simulink model "imu"  (R2013b)
settings: Solver=ode3  StartTime=0.0  StopTime=20  FixedStep=0.001  RelTol=1e-3
undefined symbols (not defined in the file or in its folder): DiscIntNeverNeededParam
libraries: simulink x1
settings Model: Creator=Ugo Pattacini  LastModifiedBy=Ugo Pattacini

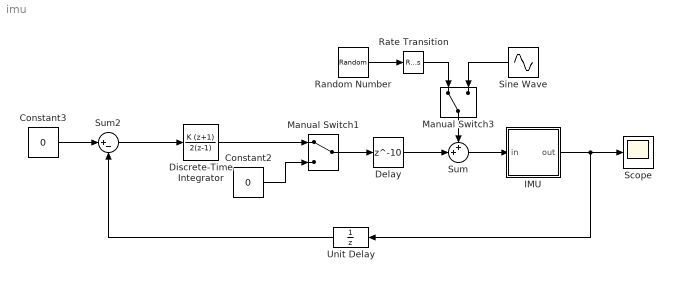
== system imu ==
  Constant2 : Constant  Value=0
  Constant3 : Constant  Value=0
  Delay : Delay  DelayLength=10  SampleTime=0.01
  Discrete-Time Integrator : DiscreteIntegrator  IntegratorMethod=Accumulation: Trapezoidal  gainval=0.05  SampleTime=0.01  ICPrevOutput=DiscIntNeverNeededParam  ICPrevScaledInput=DiscIntNeverNeededParam
  IMU : Subsystem
      mask Display: disp('IMU');
  Manual Switch1 : ManualSwitch
  Manual Switch3 : ManualSwitch
  Random Number : RandomNumber  Variance=20  SampleTime=2
  Rate Transition : RateTransition
  Scope : Scope
      settings: YMin=-20  YMax=20
  Sine Wave : Sin  Amplitude=20  Frequency=2*pi  SampleTime=0.01
  Sum : Sum  Inputs=++|  SampleTime=0.01
  Sum2 : Sum  Inputs=|+-
  Unit Delay : UnitDelay  SampleTime=-1
  wires:
  Constant2/1 -> Manual Switch1/2
  Sum2/1 -> Discrete-Time Integrator/1
  Constant3/1 -> Sum2/1
  Discrete-Time Integrator/1 -> Manual Switch1/1
  Unit Delay/1 -> Sum2/2
  Manual Switch3/1 -> Sum/1
  Random Number/1 -> Rate Transition/1
  Sine Wave/1 -> Manual Switch3/2
  Manual Switch1/1 -> Delay/1
  Delay/1 -> Sum/2
  IMU/1(out) -> Unit Delay/1, Scope/1
  Sum/1 -> IMU/1(in)
  Rate Transition/1 -> Manual Switch3/1

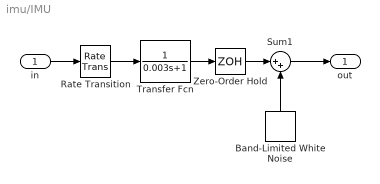
== system imu/IMU ==
  in : Inport
  Band-Limited White Noise : simulink/Sources/Band-Limited White Noise  Cov=[0.02]  Ts=0.01  seed=[23341]
  Rate Transition : RateTransition
  Sum1 : Sum  Inputs=|++
  Transfer Fcn : TransferFcn  Denominator=[0.003 1]
  Zero-Order Hold : ZeroOrderHold  SampleTime=0.01
  out : Outport
  wires:
  Zero-Order Hold/1 -> Sum1/1
  Transfer Fcn/1 -> Zero-Order Hold/1
  Sum1/1 -> out/1
  Band-Limited White Noise/1 -> Sum1/2
  Rate Transition/1 -> Transfer Fcn/1
  in/1 -> Rate Transition/1
